simulink model "UrbanPHIL"  (Simulink 8.1)
settings: Solver=ode1  StartTime=0.0  StopTime=inf  FixedStep=Ts  MaxStep=1e-3  RelTol=1e-3
PostLoadFcn:
  | NREL_Mode=1; BANSHEE_init;
InitFcn:
  | NREL_Mode=1; BANSHEE_init;
values from neighbouring files (symbols this model uses):
  Ts = 100E-6    (= 0.0001)    [BANSHEE_init.m]    (also in Ghost_init.m)
undefined symbols (not defined in the file or in its folder): Hydride, Left, Metal, Nickel, type, V
libraries: powerlib x50, rteventslib x26, rtio_opalrt_op5142ex1 x25, artemis x13, simulink x6, cables_lib x4, relay_housing_lib x3, rtlab x2, utility_service_lib x1, Feeder1_lib x1, Feeder2_lib x1, Feeder3_lib x1
(part 3 of 3)

== system UrbanPHIL/SS_PV_BESS/EPC/Inverter_Batt_RTE/TSB_hiZ snubber_free (contains 6 real diode) ==
  note: Rule of the thumb for Rsnubber=Lload/Ts
      | put maximum R for stability,
      | Then add 1-10 uf typ for Csnubber to make sure current goes to zero after a while
  g : Inport
  Demux5 : Demux  Outputs=[2 2 2]
  MMC_1P1 : Subsystem  mask(MMC cell){Ron=1e-3, Vf=0, Gp=1000/100, Gi=100*0.1e-6, Ts=Ts, dc_short_resistance=10, alt_Idc=off, alt_Idc_comp=.5}
      mask prompts: Ron "Switch conduction resistance [Ohms]"; Vf "Switch conduction voltage offset [V]"; Gp "Snubber resistance (in high impedance mode only) [Ohms]"; Gi "Snubber capacitor (in high impedance mode only) [Farads]"; Ts "Sample time [s]"; dc_short_resistance "Anti-voltage reversal equivalent diode resistance  [Ohms]"; alt_Idc "Alternate Idc calculation method based on power balance"; alt_Idc_comp "Alternate Idc compensation factor (default=0) (0...1)"
      mask help:
      | The MMC cell block implement a unipolar bridge with a capacitor.
      | Series RC snubber circuits are connected in parallel with each switch device.
      |
      | Press Help for suggested snubber values when the model is discretized.
      mask Help: eval('fts2help(''ARTEMiSMMC1PCell'');');
      mask Callback alt_Idc:
      | block=gcb;
      | x=get_param(block,'alt_Idc');
      | y=get_param(block,'MaskVisibilities');
      | if isequal (x,'on')
      |     y{8}='on';
      | else
      |     y{8}='off';
      | end
      | set_param(block,'MaskVisibilities',y);
  MMC_1P2 : Subsystem  mask(MMC cell){Ron=1e-3, Vf=0, Gp=1000/100, Gi=100*0.1e-6, Ts=Ts, dc_short_resistance=10, alt_Idc=off, alt_Idc_comp=.5}
      mask prompts: Ron "Switch conduction resistance [Ohms]"; Vf "Switch conduction voltage offset [V]"; Gp "Snubber resistance (in high impedance mode only) [Ohms]"; Gi "Snubber capacitor (in high impedance mode only) [Farads]"; Ts "Sample time [s]"; dc_short_resistance "Anti-voltage reversal equivalent diode resistance  [Ohms]"; alt_Idc "Alternate Idc calculation method based on power balance"; alt_Idc_comp "Alternate Idc compensation factor (default=0) (0...1)"
      mask help:
      | The MMC cell block implement a unipolar bridge with a capacitor.
      | Series RC snubber circuits are connected in parallel with each switch device.
      |
      | Press Help for suggested snubber values when the model is discretized.
      mask Help: eval('fts2help(''ARTEMiSMMC1PCell'');');
      mask Callback alt_Idc:
      | block=gcb;
      | x=get_param(block,'alt_Idc');
      | y=get_param(block,'MaskVisibilities');
      | if isequal (x,'on')
      |     y{8}='on';
      | else
      |     y{8}='off';
      | end
      | set_param(block,'MaskVisibilities',y);
  MMC_1P3 : Subsystem  mask(MMC cell){Ron=1e-3, Vf=0, Gp=1000/100, Gi=100*0.1e-6, Ts=Ts, dc_short_resistance=10, alt_Idc=off, alt_Idc_comp=.5}
      mask prompts: Ron "Switch conduction resistance [Ohms]"; Vf "Switch conduction voltage offset [V]"; Gp "Snubber resistance (in high impedance mode only) [Ohms]"; Gi "Snubber capacitor (in high impedance mode only) [Farads]"; Ts "Sample time [s]"; dc_short_resistance "Anti-voltage reversal equivalent diode resistance  [Ohms]"; alt_Idc "Alternate Idc calculation method based on power balance"; alt_Idc_comp "Alternate Idc compensation factor (default=0) (0...1)"
      mask help:
      | The MMC cell block implement a unipolar bridge with a capacitor.
      | Series RC snubber circuits are connected in parallel with each switch device.
      |
      | Press Help for suggested snubber values when the model is discretized.
      mask Help: eval('fts2help(''ARTEMiSMMC1PCell'');');
      mask Callback alt_Idc:
      | block=gcb;
      | x=get_param(block,'alt_Idc');
      | y=get_param(block,'MaskVisibilities');
      | if isequal (x,'on')
      |     y{8}='on';
      | else
      |     y{8}='off';
      | end
      | set_param(block,'MaskVisibilities',y);
  + : PMIOPort  Port=1  Side=Right
  A : PMIOPort  Port=2  Side=Left
  - : PMIOPort  Port=3  Side=Right
  B : PMIOPort  Port=4  Side=Left
  C : PMIOPort  Port=5  Side=Left
  wires:
  Demux5/1 -> MMC_1P1/1(g)
  Demux5/2 -> MMC_1P2/1(g)
  Demux5/3 -> MMC_1P3/1(g)
  g/1 -> Demux5/1
  connections:
  A/RConn1 -- MMC_1P1/LConn1
  B/RConn1 -- MMC_1P2/LConn1
  C/RConn1 -- MMC_1P3/LConn1
  MMC_1P3/RConn1 -- +/RConn1 -- MMC_1P1/RConn1 -- MMC_1P2/RConn1
  MMC_1P3/RConn2 -- -/RConn1 -- MMC_1P1/RConn2 -- MMC_1P2/RConn2

== system UrbanPHIL/SC_ctrl/EPC Inverter/16TSDIn/16 TSDOut GR3/Dout state ctrl/Dout_CH16_CH23 ==
  Bus Creator1 : BusCreator  Inputs=8
  Dout_CH{16..23} (8 alike) : Constant  Value=[1 0 1 0]
  Manual Switch{17..24} (8 alike) : ManualSwitch
  Zero_Dout_CH{16..23} (8 alike) : Constant  Value=[0 0 0 0]
  Dout_CH8_CH15 : Outport
  wires:
  Bus Creator1/1 -> Dout_CH8_CH15/1
  Dout_CH16/1 -> Manual Switch17/1
  Zero_Dout_CH16/1 -> Manual Switch17/2
  Dout_CH17/1 -> Manual Switch18/1
  Zero_Dout_CH17/1 -> Manual Switch18/2
  Dout_CH18/1 -> Manual Switch19/1
  Zero_Dout_CH18/1 -> Manual Switch19/2
  Dout_CH19/1 -> Manual Switch20/1
  Zero_Dout_CH19/1 -> Manual Switch20/2
  Dout_CH20/1 -> Manual Switch21/1
  Zero_Dout_CH20/1 -> Manual Switch21/2
  Dout_CH21/1 -> Manual Switch22/1
  Zero_Dout_CH21/1 -> Manual Switch22/2
  Dout_CH22/1 -> Manual Switch23/1
  Zero_Dout_CH22/1 -> Manual Switch23/2
  Dout_CH23/1 -> Manual Switch24/1
  Zero_Dout_CH23/1 -> Manual Switch24/2
  Manual Switch17/1 -> Bus Creator1/1  "states 17"
  Manual Switch18/1 -> Bus Creator1/2  "states 18"
  Manual Switch19/1 -> Bus Creator1/3  "states 19"
  Manual Switch20/1 -> Bus Creator1/4  "states 20"
  Manual Switch21/1 -> Bus Creator1/5  "states 21"
  Manual Switch22/1 -> Bus Creator1/6  "states 22"
  Manual Switch23/1 -> Bus Creator1/7  "states 23"
  Manual Switch24/1 -> Bus Creator1/8  "states 24"

== system UrbanPHIL/SC_ctrl/EPC Inverter/16TSDIn/16 TSDOut GR3/Dout state ctrl/Dout_CH24_CH31 ==
  Bus Creator : BusCreator  Inputs=8
  Dout_CH{24..31} (8 alike) : Constant  Value=[1 0 1 0]
  Manual Switch{25..32} (8 alike) : ManualSwitch
  Zero_Dout_CH{24..31} (8 alike) : Constant  Value=[0 0 0 0]
  Dout_CH8_CH15 : Outport
  wires:
  Manual Switch32/1 -> Bus Creator/8  "states 32"
  Manual Switch31/1 -> Bus Creator/7  "states 31"
  Manual Switch30/1 -> Bus Creator/6  "states 30"
  Manual Switch29/1 -> Bus Creator/5  "states 29"
  Manual Switch28/1 -> Bus Creator/4  "states 28"
  Manual Switch27/1 -> Bus Creator/3  "states 27"
  Manual Switch26/1 -> Bus Creator/2  "states 26"
  Manual Switch25/1 -> Bus Creator/1  "states 25"
  Zero_Dout_CH31/1 -> Manual Switch32/2
  Dout_CH31/1 -> Manual Switch32/1
  Zero_Dout_CH30/1 -> Manual Switch31/2
  Dout_CH30/1 -> Manual Switch31/1
  Zero_Dout_CH29/1 -> Manual Switch30/2
  Dout_CH29/1 -> Manual Switch30/1
  Zero_Dout_CH28/1 -> Manual Switch29/2
  Dout_CH28/1 -> Manual Switch29/1
  Zero_Dout_CH27/1 -> Manual Switch28/2
  Dout_CH27/1 -> Manual Switch28/1
  Zero_Dout_CH26/1 -> Manual Switch27/2
  Dout_CH26/1 -> Manual Switch27/1
  Zero_Dout_CH25/1 -> Manual Switch26/2
  Dout_CH25/1 -> Manual Switch26/1
  Zero_Dout_CH24/1 -> Manual Switch25/2
  Dout_CH24/1 -> Manual Switch25/1
  Bus Creator/1 -> Dout_CH8_CH15/1

== system UrbanPHIL/SS_PV_BESS/EPC/Controller Mapping/6-pulse RTE PWM generator (with deadtime)/Discrete Triangular-Waveform Generator ==
  Constant : Constant  Value=Vpeak
  Constant1 : Constant  Value=NumberSteps
  Constant2 : Constant  Value=Freq_used
  Fcn2 : Fcn  Expr=u[2]/u[1]
  Fcn3 : Fcn  Expr=4 *u[1] -1
  Fcn4 : Fcn  Expr=-4 *u[1] +3
  Fd1 : Constant  Value=-1
  Fd2 : Constant
  Fd4 : Constant
  Gain1 : Gain  Gain=1/2  SaturateOnIntegerOverflow=on  OutDataTypeStr=Inherit: Same as input  ParamDataTypeStr=Inherit: Same as input
  Mux5 : Mux  Inputs=2
  Product : Product  SaturateOnIntegerOverflow=on  InputSameDT=on  OutDataTypeStr=Inherit: Same as first input
  Relational Operator1 : RelationalOperator  Operator=>  InputSameDT=on
  Relational Operator2 : RelationalOperator  Operator===  InputSameDT=on
  Sum : Sum  SaturateOnIntegerOverflow=on  InputSameDT=on  OutDataTypeStr=Inherit: Same as first input
  Sum2 : Sum  Inputs=+-  SaturateOnIntegerOverflow=on  InputSameDT=on  OutDataTypeStr=Inherit: Same as first input
  Switch : Switch  Threshold=0.5  SaturateOnIntegerOverflow=on  InputSameDT=on
  Switch1 : Switch  Threshold=0.5  SaturateOnIntegerOverflow=on  InputSameDT=on
  Unit Delay : UnitDelay  SampleTime=Ts
  Unit Delay1 : UnitDelay  SampleTime=Ts
  Triangle : Outport  InitialOutput=0
  Freq_used : Outport  Port=2  InitialOutput=0
  wires:
  Constant2/1 -> Freq_used/1
  Relational Operator1/1 -> Switch1/2
  Gain1/1 -> Relational Operator1/2
  Fcn3/1 -> Switch1/3
  Fcn4/1 -> Switch1/1
  Mux5/1 -> Fcn2/1
  Fcn2/1 -> Fcn3/1, Fcn4/1
  Sum/1 -> Mux5/2, Relational Operator1/1, Relational Operator2/2, Unit Delay/1
  Constant1/1 -> Gain1/1, Mux5/1, Sum2/1
  Sum2/1 -> Relational Operator2/1
  Relational Operator2/1 -> Unit Delay1/1
  Unit Delay1/1 -> Switch/2
  Unit Delay/1 -> Switch/3
  Fd1/1 -> Switch/1
  Fd2/1 -> Sum/2
  Switch/1 -> Sum/1
  Fd4/1 -> Sum2/2
  Constant/1 -> Product/1
  Switch1/1 -> Product/2
  Product/1 -> Triangle/1

== system UrbanPHIL/SS_PV_BESS/EPC/Controller Mapping/EPC Inverter Controller Outputs/DIO - Gr4 ==
  Dout : Inport
  Bus Creator : BusCreator  Inputs=2
  Bus Selector : BusSelector  OutputSignals=DI_CH00-07  OutputAsBus=on
  Bus Selector1 : BusSelector  OutputSignals=DI_CH08-15  OutputAsBus=on
  Conditioning : Subsystem
  Conditioning1 : Subsystem
  OP5142EX2 DigitalIn : rtio_opalrt_op5142ex1/OP5142EX1 DigitalIn  CtrlName='OP5142EX2 Ctrl'  portNb=3  FcnNos=Slot 4 Module A Subsection 1  size=1  maxcount=8  count=8  sampleTime=0  numchan=8
      settings: AttributesFormatString=%<CtrlName>
  OP5142EX2 DigitalIn1 : rtio_opalrt_op5142ex1/OP5142EX1 DigitalIn  CtrlName='OP5142EX2 Ctrl'  portNb=4  FcnNos=Slot 4 Module A Subsection 2  size=1  maxcount=8  count=8  sampleTime=0  numchan=8
      settings: AttributesFormatString=%<CtrlName>
  OP5142EX2 DigitalOut : rtio_opalrt_op5142ex1/OP5142EX1 DigitalOut  CtrlName='OP5142EX2 Ctrl'  portNb=9  FcnNos=Slot 4 Module B Subsection 1  size=1  maxcount=8  count=8  numchan=8
      settings: AttributesFormatString=%<CtrlName>
  OP5142EX2 DigitalOut1 : rtio_opalrt_op5142ex1/OP5142EX1 DigitalOut  CtrlName='OP5142EX2 Ctrl'  portNb=10  FcnNos=Slot 4 Module B Subsection 2  size=1  maxcount=8  count=8  numchan=8
      settings: AttributesFormatString=%<CtrlName>
  Terminator{1,3,5..6} (4 alike) : Terminator
  DIn : Outport
  wires:
  OP5142EX2 DigitalOut/1 -> Terminator3/1
  OP5142EX2 DigitalOut1/1 -> Terminator1/1
  Dout/1 -> Bus Selector/1, Bus Selector1/1
  Bus Selector/1 -> OP5142EX2 DigitalOut/1
  Bus Selector1/1 -> OP5142EX2 DigitalOut1/1
  OP5142EX2 DigitalIn/2 -> Terminator5/1
  OP5142EX2 DigitalIn1/2 -> Terminator6/1
  OP5142EX2 DigitalIn/1 -> Conditioning/1(In1)  "DI_CH00-07"
  OP5142EX2 DigitalIn1/1 -> Conditioning1/1(In1)  "DI_CH08-15"
  Bus Creator/1 -> DIn/1
  Conditioning/1(Out1) -> Bus Creator/1
  Conditioning1/1(Out1) -> Bus Creator/2

== system UrbanPHIL/SS_PV_BESS/EPC/Controller Mapping/EPC Inverter Controller Outputs/DOUT type config ==
  note: The Constants are used to select Digital Output type:
      | - 0: Time-Stamped Digital Output
      | - 1: Pulse-Width Modulated DIgital Output
  OP5142EX2 DataIn Send : rtio_opalrt_op5142ex1/OP5142EX1 DataIn Send  CtrlName='OP5142EX2 Ctrl'  FcnNosp1=15  FcnNos=-1  FcnNosm1=(15)-1  width=1  portType=double  numwidth=1
      settings: AttributesFormatString=%<CtrlName>
  OP5142EX2 DataIn Send1 : rtio_opalrt_op5142ex1/OP5142EX1 DataIn Send  CtrlName='OP5142EX2 Ctrl'  FcnNosp1=16  FcnNos=-1  FcnNosm1=(16)-1  width=1  portType=double  numwidth=1
      settings: AttributesFormatString=%<CtrlName>
  Subsection 3 DOUT type : Constant  Value=0
  Subsection 4 DOUT type : Constant  Value=0
  Terminator1 : Terminator
  Terminator2 : Terminator
  wires:
  Subsection 3 DOUT type/1 -> OP5142EX2 DataIn Send/1
  Subsection 4 DOUT type/1 -> OP5142EX2 DataIn Send1/1
  OP5142EX2 DataIn Send1/1 -> Terminator1/1
  OP5142EX2 DataIn Send/1 -> Terminator2/1

== system UrbanPHIL/SS_PV_BESS/EPC/Controller Mapping/EPC Inverter Controller Outputs/GR1 B AIN (CH00-15) ==
  Mux6 : Mux  Inputs=2
  OP5142EX2 AnalogIn : rtio_opalrt_op5142ex1/OP5142EX1 AnalogIn  CtrlName='OP5142EX2 Ctrl'  portNb=1  FcnNos=Slot 1 Module B Subsection 1  size=16  maxcount=8  count=8  numchan=8  sampleTime=0
      settings: AttributesFormatString=%<CtrlName>
  OP5142EX2 AnalogIn1 : rtio_opalrt_op5142ex1/OP5142EX1 AnalogIn  CtrlName='OP5142EX2 Ctrl'  portNb=2  FcnNos=Slot 1 Module B Subsection 2  size=16  maxcount=8  count=8  numchan=8  sampleTime=0
      settings: AttributesFormatString=%<CtrlName>
  Terminator2 : Terminator
  Terminator3 : Terminator
  Ain : Outport
  wires:
  Mux6/1 -> Ain/1
  OP5142EX2 AnalogIn1/2 -> Terminator3/1
  OP5142EX2 AnalogIn/2 -> Terminator2/1
  OP5142EX2 AnalogIn1/1 -> Mux6/2
  OP5142EX2 AnalogIn/1 -> Mux6/1

== system UrbanPHIL/SS_PV_BESS/EPC/Controller Mapping/EPC Inverter Controller Outputs/PWM IO - Gr4 ==
  PWMOut : Inport
  Bus Creator : BusCreator  Inputs=2
  Bus Creator1 : BusCreator  Inputs=2
  Bus Creator2 : BusCreator  Inputs=2
  Bus Selector : BusSelector  OutputSignals=FreqPWMOut16-23,DutyPWMOut16-23
  Bus Selector1 : BusSelector  OutputSignals=FreqPWMOut24-31,DutyPWMOut24-31
  Bus Selector2 : BusSelector  OutputSignals=Ch16-23,Ch24-31
  OP5142EX2 PWM In : rtio_opalrt_op5142ex1/OP5142EX1 PWM In  CtrlName='OP5142EX2 Ctrl'  portNb=7  FcnNos=Slot 4 Module A Subsection 3  maxCount=8  Count=8  sampleTime=0  numchan=8
      settings: AttributesFormatString=%<CtrlName>
  OP5142EX2 PWM In1 : rtio_opalrt_op5142ex1/OP5142EX1 PWM In  CtrlName='OP5142EX2 Ctrl'  portNb=8  FcnNos=Slot 4 Module A Subsection 4  maxCount=8  Count=8  sampleTime=0  numchan=8
      settings: AttributesFormatString=%<CtrlName>
  OP5142EX2 PWM Out : rtio_opalrt_op5142ex1/OP5142EX1 PWM Out  CtrlName='OP5142EX2 Ctrl'  portNb=13  FcnNos=Slot 4 Module B Subsection 3  size=64  maxcount=8  count=8  polarity=Active High  symMode=Symmetric  complementary=off  deadTime=0  numchan=8  loadnb=1  initphase=[0 0 0 0 0 0 0 0]  dutyhalf=At each PWM period
      settings: AttributesFormatString=%<CtrlName>
  OP5142EX2 PWM Out1 : rtio_opalrt_op5142ex1/OP5142EX1 PWM Out  CtrlName='OP5142EX2 Ctrl'  portNb=14  FcnNos=Slot 4 Module B Subsection 4  size=64  maxcount=8  count=8  polarity=Active High  symMode=Symmetric  complementary=off  deadTime=0  numchan=8  loadnb=2  initphase=[0 0 0 0 0 0 0 0]  dutyhalf=At each PWM period
      settings: AttributesFormatString=%<CtrlName>
  RTE PWM Top 1 : rteventslib/Sources/RTE PWM  ShiftedTransition=Enabled  MaxEvents=4  SampleTime=Ts
  Terminator{,1,4..5} (4 alike) : Terminator
  PWMIn : Outport
  PWMIn_RTE : Outport  Port=2
  wires:
  Bus Selector/1 -> OP5142EX2 PWM Out/1  "<FreqPWMOut16-23>"
  Bus Selector/2 -> OP5142EX2 PWM Out/2  "<DutyPWMOut16-23>"
  OP5142EX2 PWM Out/1 -> Terminator/1
  Bus Selector1/1 -> OP5142EX2 PWM Out1/1  "<FreqPWMOut24-31>"
  Bus Selector1/2 -> OP5142EX2 PWM Out1/2  "<DutyPWMOut24-31>"
  OP5142EX2 PWM Out1/1 -> Terminator1/1
  PWMOut/1 -> Bus Selector2/1
  Bus Selector2/1 -> Bus Selector/1  "<Ch16-23>"
  Bus Creator/1 -> PWMIn/1
  Bus Creator1/1 -> Bus Creator/1  "PWMI_CH16-23"
  Bus Creator2/1 -> Bus Creator/2  "PWMI_CH24-31"
  OP5142EX2 PWM In1/3 -> Terminator5/1
  OP5142EX2 PWM In/3 -> Terminator4/1
  OP5142EX2 PWM In/1 -> Bus Creator1/1, RTE PWM Top 1/1  "Freq"
  OP5142EX2 PWM In/2 -> Bus Creator1/2, RTE PWM Top 1/2  "Duty"
  OP5142EX2 PWM In1/1 -> Bus Creator2/1  "Freq"
  OP5142EX2 PWM In1/2 -> Bus Creator2/2  "Duty"
  Bus Selector2/2 -> Bus Selector1/1  "<Ch24-31>"
  RTE PWM Top 1/1 -> PWMIn_RTE/1

== system UrbanPHIL/SS_PV_BESS/EPC/Controller Mapping/EPC Inverter Controller Outputs/TSDIO - Gr4 ==
  note: States
      | Times
      | for each channel
      |
      | Status for the block.
  TSDout : Inport
  Bus Creator : BusCreator  Inputs=16
  Bus Creator1 : BusCreator  Inputs=16
  Bus Creator2 : BusCreator  Inputs=2
  Bus Selector : BusSelector  OutputSignals=states.CH16-23.states 17,times CH16-23.times17,states.CH16-23.states 18,times CH16-23.times18,states.CH16-23.states 19,times CH16-23.times19,states.CH16-23.states 20,times CH16-23.times20,states.CH16-23.states 21,times CH16-23.times21,states.CH16-23.states 22,times CH16-23.times22,states.CH16-23.states 23,times CH16-23.times23,states.CH16-23.states 24,times CH16-23.times24
  Bus Selector1 : BusSelector  OutputSignals=states.CH24-31.states 25,times CH24-31.times25,states.CH24-31.states 26,times CH24-31.times26,states.CH24-31.states 27,times CH24-31.times27,states.CH24-31.states 28,times CH24-31.times28,states.CH24-31.states 29,times CH24-31.times29,states.CH24-31.states 30,times CH24-31.times30,states.CH24-31.states 31,times CH24-31.times31,states.CH24-31.states 32,times CH24-31.times32
  Bus Selector2 : BusSelector  OutputSignals=states1,times1,states2,times2,states3,times3,states4,times4,states5,times5,states6,times6
  OP5142EX2 EventDetector : rtio_opalrt_op5142ex1/OP5142EX1 EventDetector  CtrlName='OP5142EX2 Ctrl'  portNb=5  FcnNos=Slot 4 Module A Subsection 3  size=32  count=8  nbChannels=8  width=4  timeUnit=Time ratio  sampleTime=0  numwidth=4
      settings: AttributesFormatString=%<CtrlName>
  OP5142EX2 EventDetector1 : rtio_opalrt_op5142ex1/OP5142EX1 EventDetector  CtrlName='OP5142EX2 Ctrl'  portNb=6  FcnNos=Slot 4 Module A Subsection 4  size=32  count=8  nbChannels=8  width=4  timeUnit=Time ratio  sampleTime=0  numwidth=4
      settings: AttributesFormatString=%<CtrlName>
  OP5142EX2 EventGenerator : rtio_opalrt_op5142ex1/OP5142EX1 EventGenerator  CtrlName='OP5142EX2 Ctrl'  portNb=11  FcnNos=Slot 4 Module B Subsection 3  size=32  count=8  nbChannels=8  width=4  timeUnit=Time ratio  numwidth=4
      settings: AttributesFormatString=%<CtrlName>
  OP5142EX2 EventGenerator1 : rtio_opalrt_op5142ex1/OP5142EX1 EventGenerator  CtrlName='OP5142EX2 Ctrl'  portNb=12  FcnNos=Slot 4 Module B Subsection 4  size=32  count=8  nbChannels=8  width=4  timeUnit=Time ratio  numwidth=4
      settings: AttributesFormatString=%<CtrlName>
  RTE Conversion OP5110-5120 Event Generator/Detector : rteventslib/Signal Attributes/RTE Conversion OP5110-5120 Event Generator//Detector  conversionType=OP5110-5120 to RTE Boolean  nbLine=6  nbEvents=4  timeUnit=Time Ratio  enTimeFactor=off  sampleTime=Ts  initStates=off
  Terminator{,1..3} (4 alike) : Terminator
  TSDin : Outport
  TSDin_RTE : Outport  Port=2
  wires:
  TSDout/1 -> Bus Selector/1, Bus Selector1/1
  Bus Selector/16 -> OP5142EX2 EventGenerator/16  "<times24>"
  Bus Selector/15 -> OP5142EX2 EventGenerator/15  "<states 24>"
  Bus Selector/14 -> OP5142EX2 EventGenerator/14  "<times23>"
  Bus Selector/13 -> OP5142EX2 EventGenerator/13  "<states 23>"
  Bus Selector/12 -> OP5142EX2 EventGenerator/12  "<times22>"
  Bus Selector/11 -> OP5142EX2 EventGenerator/11  "<states 22>"
  Bus Selector/10 -> OP5142EX2 EventGenerator/10  "<times21>"
  Bus Selector/9 -> OP5142EX2 EventGenerator/9  "<states 21>"
  Bus Selector/8 -> OP5142EX2 EventGenerator/8  "<times20>"
  Bus Selector/7 -> OP5142EX2 EventGenerator/7  "<states 20>"
  Bus Selector/6 -> OP5142EX2 EventGenerator/6  "<times19>"
  Bus Selector/5 -> OP5142EX2 EventGenerator/5  "<states 19>"
  Bus Selector/4 -> OP5142EX2 EventGenerator/4  "<times18>"
  Bus Selector/3 -> OP5142EX2 EventGenerator/3  "<states 18>"
  Bus Selector/2 -> OP5142EX2 EventGenerator/2  "<times17>"
  Bus Selector/1 -> OP5142EX2 EventGenerator/1  "<states 17>"
  OP5142EX2 EventGenerator/1 -> Terminator/1
  OP5142EX2 EventDetector/16 -> Bus Creator/16  "times8"
  OP5142EX2 EventDetector/15 -> Bus Creator/15  "states8"
  OP5142EX2 EventDetector/14 -> Bus Creator/14  "times7"
  OP5142EX2 EventDetector/13 -> Bus Creator/13  "states7"
  OP5142EX2 EventDetector/12 -> Bus Creator/12  "times6"
  OP5142EX2 EventDetector/11 -> Bus Creator/11  "states6"
  OP5142EX2 EventDetector/10 -> Bus Creator/10  "times5"
  OP5142EX2 EventDetector/9 -> Bus Creator/9  "states5"
  OP5142EX2 EventDetector/8 -> Bus Creator/8  "times4"
  OP5142EX2 EventDetector/7 -> Bus Creator/7  "states4"
  OP5142EX2 EventDetector/6 -> Bus Creator/6  "times3"
  OP5142EX2 EventDetector/5 -> Bus Creator/5  "states3"
  OP5142EX2 EventDetector/4 -> Bus Creator/4  "times2"
  OP5142EX2 EventDetector/3 -> Bus Creator/3  "states2"
  OP5142EX2 EventDetector/2 -> Bus Creator/2  "times1"
  OP5142EX2 EventDetector/1 -> Bus Creator/1  "states1"
  OP5142EX2 EventDetector/17 -> Terminator1/1, [status]
  OP5142EX2 EventGenerator1/1 -> Terminator2/1
  Bus Selector1/1 -> OP5142EX2 EventGenerator1/1  "<states 25>"
  Bus Selector1/2 -> OP5142EX2 EventGenerator1/2  "<times25>"
  Bus Selector1/3 -> OP5142EX2 EventGenerator1/3  "<states 26>"
  Bus Selector1/4 -> OP5142EX2 EventGenerator1/4  "<times26>"
  Bus Selector1/5 -> OP5142EX2 EventGenerator1/5  "<states 27>"
  Bus Selector1/6 -> OP5142EX2 EventGenerator1/6  "<times27>"
  Bus Selector1/7 -> OP5142EX2 EventGenerator1/7  "<states 28>"
  Bus Selector1/8 -> OP5142EX2 EventGenerator1/8  "<times28>"
  Bus Selector1/9 -> OP5142EX2 EventGenerator1/9  "<states 29>"
  Bus Selector1/10 -> OP5142EX2 EventGenerator1/10  "<times29>"
  Bus Selector1/11 -> OP5142EX2 EventGenerator1/11  "<states 30>"
  Bus Selector1/12 -> OP5142EX2 EventGenerator1/12  "<times30>"
  Bus Selector1/13 -> OP5142EX2 EventGenerator1/13  "<states 31>"
  Bus Selector1/14 -> OP5142EX2 EventGenerator1/14  "<times31>"
  Bus Selector1/15 -> OP5142EX2 EventGenerator1/15  "<states 32>"
  Bus Selector1/16 -> OP5142EX2 EventGenerator1/16  "<times32>"
  Bus Creator1/1 -> Bus Creator2/2  "CH24-31"
  OP5142EX2 EventDetector1/16 -> Bus Creator1/16  "times6"
  OP5142EX2 EventDetector1/15 -> Bus Creator1/15  "states6"
  OP5142EX2 EventDetector1/14 -> Bus Creator1/14  "times5"
  OP5142EX2 EventDetector1/13 -> Bus Creator1/13  "states5"
  OP5142EX2 EventDetector1/12 -> Bus Creator1/12  "times4"
  OP5142EX2 EventDetector1/11 -> Bus Creator1/11  "states4"
  OP5142EX2 EventDetector1/10 -> Bus Creator1/10  "times3"
  OP5142EX2 EventDetector1/9 -> Bus Creator1/9  "states3"
  OP5142EX2 EventDetector1/8 -> Bus Creator1/8  "times2"
  OP5142EX2 EventDetector1/7 -> Bus Creator1/7  "states2"
  OP5142EX2 EventDetector1/6 -> Bus Creator1/6  "times1"
  OP5142EX2 EventDetector1/5 -> Bus Creator1/5  "states1"
  OP5142EX2 EventDetector1/4 -> Bus Creator1/4  "times2"
  OP5142EX2 EventDetector1/3 -> Bus Creator1/3  "states2"
  OP5142EX2 EventDetector1/2 -> Bus Creator1/2  "times1"
  OP5142EX2 EventDetector1/1 -> Bus Creator1/1  "states1"
  OP5142EX2 EventDetector1/17 -> Terminator3/1  "states7"
  Bus Creator/1 -> Bus Creator2/1, Bus Selector2/1  "CH16-23"
  Bus Creator2/1 -> TSDin/1  "TSDIN"
  Bus Selector2/1 -> RTE Conversion OP5110-5120 Event Generator/Detector/1  "<states1>"
  Bus Selector2/3 -> RTE Conversion OP5110-5120 Event Generator/Detector/4  "<states2>"
  [status] -> RTE Conversion OP5110-5120 Event Generator/Detector/3
  [status] -> RTE Conversion OP5110-5120 Event Generator/Detector/6
  Bus Selector2/5 -> RTE Conversion OP5110-5120 Event Generator/Detector/7  "<states3>"
  Bus Selector2/2 -> RTE Conversion OP5110-5120 Event Generator/Detector/2  "<times1>"
  Bus Selector2/4 -> RTE Conversion OP5110-5120 Event Generator/Detector/5  "<times2>"
  Bus Selector2/6 -> RTE Conversion OP5110-5120 Event Generator/Detector/8  "<times3>"
  [status] -> RTE Conversion OP5110-5120 Event Generator/Detector/9
  Bus Selector2/7 -> RTE Conversion OP5110-5120 Event Generator/Detector/10  "<states4>"
  Bus Selector2/8 -> RTE Conversion OP5110-5120 Event Generator/Detector/11  "<times4>"
  [status] -> RTE Conversion OP5110-5120 Event Generator/Detector/12
  Bus Selector2/9 -> RTE Conversion OP5110-5120 Event Generator/Detector/13  "<states5>"
  Bus Selector2/10 -> RTE Conversion OP5110-5120 Event Generator/Detector/14  "<times5>"
  [status] -> RTE Conversion OP5110-5120 Event Generator/Detector/15
  Bus Selector2/11 -> RTE Conversion OP5110-5120 Event Generator/Detector/16  "<states6>"
  Bus Selector2/12 -> RTE Conversion OP5110-5120 Event Generator/Detector/17  "<times6>"
  [status] -> RTE Conversion OP5110-5120 Event Generator/Detector/18
  RTE Conversion OP5110-5120 Event Generator/Detector/1 -> TSDin_RTE/1

== system UrbanPHIL/SS_PV_BESS/EPC/Inverter_Batt_RTE/TSB_hiZ snubber_free (contains 6 real diode)/MMC_1P1 ==
  g : Inport
  Constant2 : Constant  Value=Ts
  Constant9 : Constant  Value=0
  Controlled Current Source : powerlib/Electrical Sources/Controlled Current Source  Initialize=on  Source_Type=AC  Amplitude=0  Phase=0  Frequency=0  Measurements=None
  Demux1 : Demux  Outputs=2
  Diode : powerlib/Power Electronics/Diode  Ron=Ron  Lon=0  Vf=0  IC=0  UseSnubber=off  Rs=Gp  Cs=Gi  Measurements=off
  Diode1 : powerlib/Power Electronics/Diode  Ron=Ron  Lon=0  Vf=0  IC=0  UseSnubber=off  Rs=Gp  Cs=Gi  Measurements=off
  IMeasure_1 : powerlib/Measurements/Current Measurement  PhasorSimulation=off  OutputType=Magnitude  PSBequivalent=0
  IMeasure_2 : powerlib/Measurements/Current Measurement  PhasorSimulation=off  OutputType=Magnitude  PSBequivalent=0
  MMC_cell_Sfunction : Subsystem
  Memory1 : Memory  InheritSampleTime=on
  Memory2 : Memory  InheritSampleTime=on
  Memory4 : Memory  InheritSampleTime=on
  Switch1 : Switch  Threshold=0.5
  Switch2 : Switch  Threshold=0.5
  Switch4 : Switch  Threshold=0.5
  VSource_2 : powerlib/Electrical Sources/Controlled Voltage Source  Initialize=off  Source_Type=AC  Amplitude=0  Phase=0  Frequency=0  Measurements=None
  VSource_3 : powerlib/Electrical Sources/Controlled Voltage Source  Initialize=off  Source_Type=AC  Amplitude=0  Phase=0  Frequency=0  Measurements=None
  Voltage Measurement : powerlib/Measurements/Voltage Measurement  PhasorSimulation=off  OutputType=Complex  PSBequivalent=0
  A : PMIOPort  Port=1  Side=Left
  Dc+ : PMIOPort  Port=2  Side=Right
  Dc- : PMIOPort  Port=3  Side=Right
  wires:
  g/1 -> Demux1/1
  Demux1/2 -> MMC_cell_Sfunction/2(g1)
  Demux1/1 -> MMC_cell_Sfunction/1(g)
  Constant2/1 -> MMC_cell_Sfunction/3(Ts)
  MMC_cell_Sfunction/2(Vac) -> Switch4/3, Switch1/3
  IMeasure_1/1 -> Memory1/1
  Voltage Measurement/1 -> Memory4/1
  Switch4/1 -> VSource_2/1
  Switch1/1 -> VSource_3/1
  MMC_cell_Sfunction/3(hiZ) -> Switch4/2, Switch1/2, Switch2/2
  Constant9/1 -> Switch4/1
  Memory1/1 -> MMC_cell_Sfunction/4(Iac)
  Memory4/1 -> MMC_cell_Sfunction/5(Vdc), Switch1/1
  Switch2/1 -> Controlled Current Source/1
  MMC_cell_Sfunction/1(Idc) -> Switch2/3
  IMeasure_2/1 -> Memory2/1
  Memory2/1 -> Switch2/1
  connections:
  Controlled Current Source/RConn1 -- Dc-/RConn1 -- Voltage Measurement/LConn2 -- VSource_3/LConn1 -- VSource_2/LConn1
  Dc+/RConn1 -- Voltage Measurement/LConn1 -- Controlled Current Source/LConn1
  Diode1/LConn1 -- VSource_2/RConn1
  Diode1/RConn1 -- Diode/LConn1 -- IMeasure_1/LConn1
  IMeasure_1/RConn1 -- A/RConn1
  VSource_3/RConn1 -- IMeasure_2/LConn1
  IMeasure_2/RConn1 -- Diode/RConn1

== system UrbanPHIL/SS_PV_BESS/EPC/Inverter_Batt_RTE/TSB_hiZ snubber_free (contains 6 real diode)/MMC_1P2 ==
  g : Inport
  Constant2 : Constant  Value=Ts
  Constant9 : Constant  Value=0
  Controlled Current Source : powerlib/Electrical Sources/Controlled Current Source  Initialize=on  Source_Type=AC  Amplitude=0  Phase=0  Frequency=0  Measurements=None
  Demux1 : Demux  Outputs=2
  Diode : powerlib/Power Electronics/Diode  Ron=Ron  Lon=0  Vf=0  IC=0  UseSnubber=off  Rs=Gp  Cs=Gi  Measurements=off
  Diode1 : powerlib/Power Electronics/Diode  Ron=Ron  Lon=0  Vf=0  IC=0  UseSnubber=off  Rs=Gp  Cs=Gi  Measurements=off
  IMeasure_1 : powerlib/Measurements/Current Measurement  PhasorSimulation=off  OutputType=Magnitude  PSBequivalent=0
  IMeasure_2 : powerlib/Measurements/Current Measurement  PhasorSimulation=off  OutputType=Magnitude  PSBequivalent=0
  MMC_cell_Sfunction : Subsystem
  Memory1 : Memory  InheritSampleTime=on
  Memory2 : Memory  InheritSampleTime=on
  Memory4 : Memory  InheritSampleTime=on
  Switch1 : Switch  Threshold=0.5
  Switch2 : Switch  Threshold=0.5
  Switch4 : Switch  Threshold=0.5
  VSource_2 : powerlib/Electrical Sources/Controlled Voltage Source  Initialize=off  Source_Type=AC  Amplitude=0  Phase=0  Frequency=0  Measurements=None
  VSource_3 : powerlib/Electrical Sources/Controlled Voltage Source  Initialize=off  Source_Type=AC  Amplitude=0  Phase=0  Frequency=0  Measurements=None
  Voltage Measurement : powerlib/Measurements/Voltage Measurement  PhasorSimulation=off  OutputType=Complex  PSBequivalent=0
  A : PMIOPort  Port=1  Side=Left
  Dc+ : PMIOPort  Port=2  Side=Right
  Dc- : PMIOPort  Port=3  Side=Right
  wires:
  Memory2/1 -> Switch2/1
  IMeasure_2/1 -> Memory2/1
  MMC_cell_Sfunction/1(Idc) -> Switch2/3
  Switch2/1 -> Controlled Current Source/1
  Memory4/1 -> Switch1/1, MMC_cell_Sfunction/5(Vdc)
  Memory1/1 -> MMC_cell_Sfunction/4(Iac)
  Constant9/1 -> Switch4/1
  MMC_cell_Sfunction/3(hiZ) -> Switch2/2, Switch1/2, Switch4/2
  Switch1/1 -> VSource_3/1
  Switch4/1 -> VSource_2/1
  Voltage Measurement/1 -> Memory4/1
  IMeasure_1/1 -> Memory1/1
  MMC_cell_Sfunction/2(Vac) -> Switch1/3, Switch4/3
  Constant2/1 -> MMC_cell_Sfunction/3(Ts)
  Demux1/1 -> MMC_cell_Sfunction/1(g)
  Demux1/2 -> MMC_cell_Sfunction/2(g1)
  g/1 -> Demux1/1
  connections:
  IMeasure_2/RConn1 -- Diode/RConn1
  VSource_3/RConn1 -- IMeasure_2/LConn1
  IMeasure_1/RConn1 -- A/RConn1
  IMeasure_1/LConn1 -- Diode/LConn1 -- Diode1/RConn1
  Diode1/LConn1 -- VSource_2/RConn1
  Controlled Current Source/LConn1 -- Voltage Measurement/LConn1 -- Dc+/RConn1
  VSource_2/LConn1 -- VSource_3/LConn1 -- Voltage Measurement/LConn2 -- Dc-/RConn1 -- Controlled Current Source/RConn1

== system UrbanPHIL/SS_PV_BESS/EPC/Inverter_Batt_RTE/TSB_hiZ snubber_free (contains 6 real diode)/MMC_1P3 ==
  g : Inport
  Constant2 : Constant  Value=Ts
  Constant9 : Constant  Value=0
  Controlled Current Source : powerlib/Electrical Sources/Controlled Current Source  Initialize=on  Source_Type=AC  Amplitude=0  Phase=0  Frequency=0  Measurements=None
  Demux1 : Demux  Outputs=2
  Diode : powerlib/Power Electronics/Diode  Ron=Ron  Lon=0  Vf=0  IC=0  UseSnubber=off  Rs=Gp  Cs=Gi  Measurements=off
  Diode1 : powerlib/Power Electronics/Diode  Ron=Ron  Lon=0  Vf=0  IC=0  UseSnubber=off  Rs=Gp  Cs=Gi  Measurements=off
  IMeasure_1 : powerlib/Measurements/Current Measurement  PhasorSimulation=off  OutputType=Magnitude  PSBequivalent=0
  IMeasure_2 : powerlib/Measurements/Current Measurement  PhasorSimulation=off  OutputType=Magnitude  PSBequivalent=0
  MMC_cell_Sfunction : Subsystem
  Memory1 : Memory  InheritSampleTime=on
  Memory2 : Memory  InheritSampleTime=on
  Memory4 : Memory  InheritSampleTime=on
  Switch1 : Switch  Threshold=0.5
  Switch2 : Switch  Threshold=0.5
  Switch4 : Switch  Threshold=0.5
  VSource_2 : powerlib/Electrical Sources/Controlled Voltage Source  Initialize=off  Source_Type=AC  Amplitude=0  Phase=0  Frequency=0  Measurements=None
  VSource_3 : powerlib/Electrical Sources/Controlled Voltage Source  Initialize=off  Source_Type=AC  Amplitude=0  Phase=0  Frequency=0  Measurements=None
  Voltage Measurement : powerlib/Measurements/Voltage Measurement  PhasorSimulation=off  OutputType=Complex  PSBequivalent=0
  A : PMIOPort  Port=1  Side=Left
  Dc+ : PMIOPort  Port=2  Side=Right
  Dc- : PMIOPort  Port=3  Side=Right
  wires:
  g/1 -> Demux1/1
  Demux1/2 -> MMC_cell_Sfunction/2(g1)
  Demux1/1 -> MMC_cell_Sfunction/1(g)
  Constant2/1 -> MMC_cell_Sfunction/3(Ts)
  MMC_cell_Sfunction/2(Vac) -> Switch4/3, Switch1/3
  IMeasure_1/1 -> Memory1/1
  Voltage Measurement/1 -> Memory4/1
  Switch4/1 -> VSource_2/1
  Switch1/1 -> VSource_3/1
  MMC_cell_Sfunction/3(hiZ) -> Switch4/2, Switch1/2, Switch2/2
  Constant9/1 -> Switch4/1
  Memory1/1 -> MMC_cell_Sfunction/4(Iac)
  Memory4/1 -> MMC_cell_Sfunction/5(Vdc), Switch1/1
  Switch2/1 -> Controlled Current Source/1
  MMC_cell_Sfunction/1(Idc) -> Switch2/3
  IMeasure_2/1 -> Memory2/1
  Memory2/1 -> Switch2/1
  connections:
  Controlled Current Source/RConn1 -- Dc-/RConn1 -- Voltage Measurement/LConn2 -- VSource_3/LConn1 -- VSource_2/LConn1
  Dc+/RConn1 -- Voltage Measurement/LConn1 -- Controlled Current Source/LConn1
  Diode1/LConn1 -- VSource_2/RConn1
  Diode1/RConn1 -- Diode/LConn1 -- IMeasure_1/LConn1
  IMeasure_1/RConn1 -- A/RConn1
  VSource_3/RConn1 -- IMeasure_2/LConn1
  IMeasure_2/RConn1 -- Diode/RConn1

== system UrbanPHIL/SS_PV_BESS/EPC/Controller Mapping/EPC Inverter Controller Outputs/DIO - Gr4/Conditioning ==
  In1 : Inport
  Bus Creator : BusCreator  Inputs=8
  Demux : Demux  Outputs=8
  Out1 : Outport
  wires:
  Demux/1 -> Bus Creator/1  "K2_Main_DC"
  Demux/2 -> Bus Creator/2  "K1_Precharge_DC"
  Demux/3 -> Bus Creator/3  "MX2_Remote_AC"
  Demux/4 -> Bus Creator/4  "MX1_Main_AC"
  Demux/5 -> Bus Creator/5
  Demux/6 -> Bus Creator/6
  Demux/7 -> Bus Creator/7
  Demux/8 -> Bus Creator/8
  Bus Creator/1 -> Out1/1  "DI_CH00-07"
  In1/1 -> Demux/1

== system UrbanPHIL/SS_PV_BESS/EPC/Controller Mapping/EPC Inverter Controller Outputs/DIO - Gr4/Conditioning1 ==
  In1 : Inport
  Bus Creator : BusCreator  Inputs=8
  Demux : Demux  Outputs=8
  Out1 : Outport
  wires:
  In1/1 -> Demux/1
  Bus Creator/1 -> Out1/1  "DI_CH08-15"
  Demux/8 -> Bus Creator/8
  Demux/7 -> Bus Creator/7
  Demux/6 -> Bus Creator/6
  Demux/5 -> Bus Creator/5
  Demux/4 -> Bus Creator/4
  Demux/3 -> Bus Creator/3
  Demux/2 -> Bus Creator/2
  Demux/1 -> Bus Creator/1

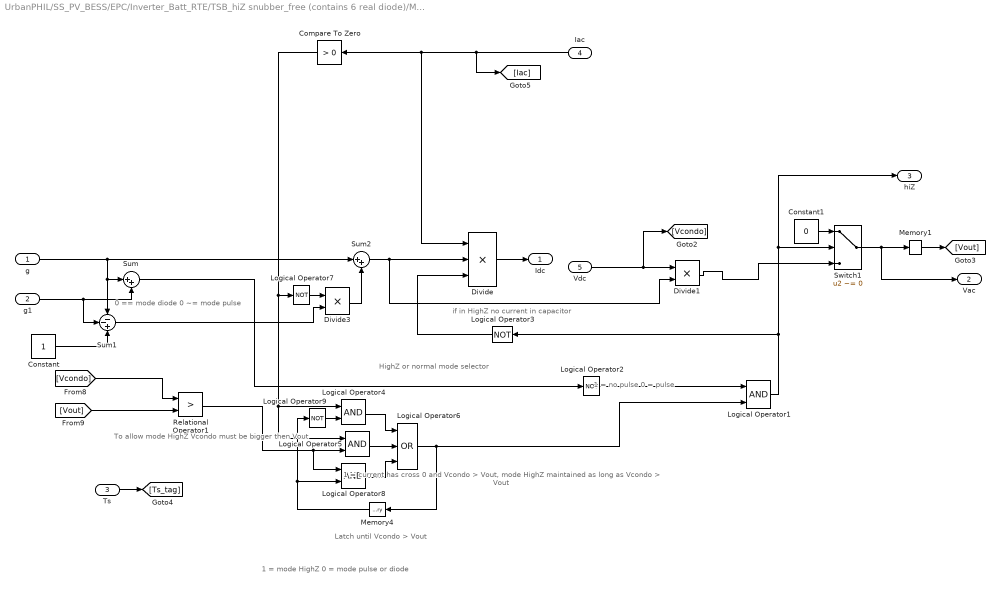
== system UrbanPHIL/SS_PV_BESS/EPC/Inverter_Batt_RTE/TSB_hiZ snubber_free (contains 6 real diode)/MMC_1P1/MMC_cell_Sfunction ==
  note: Latch until Vcondo > Vout
  note: 1 = mode HighZ
      | 0 = mode pulse or diode
  note: if in HighZ no current in capacitor
  note: 0 == mode diode
      | 0 ~= mode pulse
  note: 1 = current has cross 0 and
      | Vcondo > Vout, mode HighZ
      | maintained as long as Vcondo > Vout
  note: 1 = no pulse
      | 0 = pulse
  note: To allow mode HighZ
      | Vcondo must be bigger then
      | Vout
  note: HighZ or normal mode selector
  g : Inport
  g1 : Inport  Port=2
  Ts : Inport  Port=3
  Iac : Inport  Port=4
  Vdc : Inport  Port=5
  Compare To Zero : simulink/Logic and Bit Operations/Compare To Zero  relop=>  OutDataTypeStr=uint8
  Constant : Constant
  Constant1 : Constant  Value=0
  Divide : Product  Inputs=3
  Divide1 : Product
  Divide3 : Product
  Logical Operator{1,4..5,8} (4 alike) : Logic  AllPortsSameDT=off  OutDataTypeStr=boolean
  Logical Operator{2..3,7,9} (4 alike) : Logic  Operator=NOT  AllPortsSameDT=off  OutDataTypeStr=boolean
  Logical Operator6 : Logic  Operator=OR  Inputs=3  AllPortsSameDT=off  OutDataTypeStr=boolean
  Memory1 : Memory  InheritSampleTime=on
  Memory4 : Memory  InheritSampleTime=on
  Relational Operator1 : RelationalOperator  Operator=>  OutDataTypeStr=boolean
  Sum : Sum  Inputs=|++
  Sum1 : Sum  Inputs=--+
  Sum2 : Sum  Inputs=|++
  Switch1 : Switch  Criteria=u2 ~= 0
  Idc : Outport
  Vac : Outport  Port=2
  hiZ : Outport  Port=3
  wires:
  Memory1/1 -> [Vout]
  Divide3/1 -> Sum2/2
  Sum1/1 -> Divide3/2
  Constant/1 -> Sum1/3
  Logical Operator6/1 -> Memory4/1, Logical Operator1/2
  Logical Operator8/1 -> Logical Operator6/3
  Logical Operator5/1 -> Logical Operator6/2
  Logical Operator4/1 -> Logical Operator6/1
  Logical Operator9/1 -> Logical Operator4/2
  Relational Operator1/1 -> Logical Operator8/1, Logical Operator5/2
  Logical Operator7/1 -> Divide3/1
  Ts/1 -> [Ts_tag]
  g1/1 -> Sum1/2, Sum/2
  Logical Operator1/1 -> Logical Operator3/1, Switch1/2, hiZ/1
  [Vcondo] -> Relational Operator1/1
  Logical Operator3/1 -> Divide/3
  Logical Operator2/1 -> Logical Operator1/1
  [Vout] -> Relational Operator1/2
  Vdc/1 -> Divide1/1, [Vcondo]
  Iac/1 -> Compare To Zero/1, Divide/1, [Iac]
  Divide/1 -> Idc/1
  Compare To Zero/1 -> Logical Operator4/1, Logical Operator5/1, Logical Operator7/1
  Sum/1 -> Logical Operator2/1
  g/1 -> Sum1/1, Sum/1, Sum2/1
  Sum2/1 -> Divide1/2, Divide/2
  Divide1/1 -> Switch1/3
  Switch1/1 -> Memory1/1, Vac/1
  Memory4/1 -> Logical Operator8/2, Logical Operator9/1
  Constant1/1 -> Switch1/1

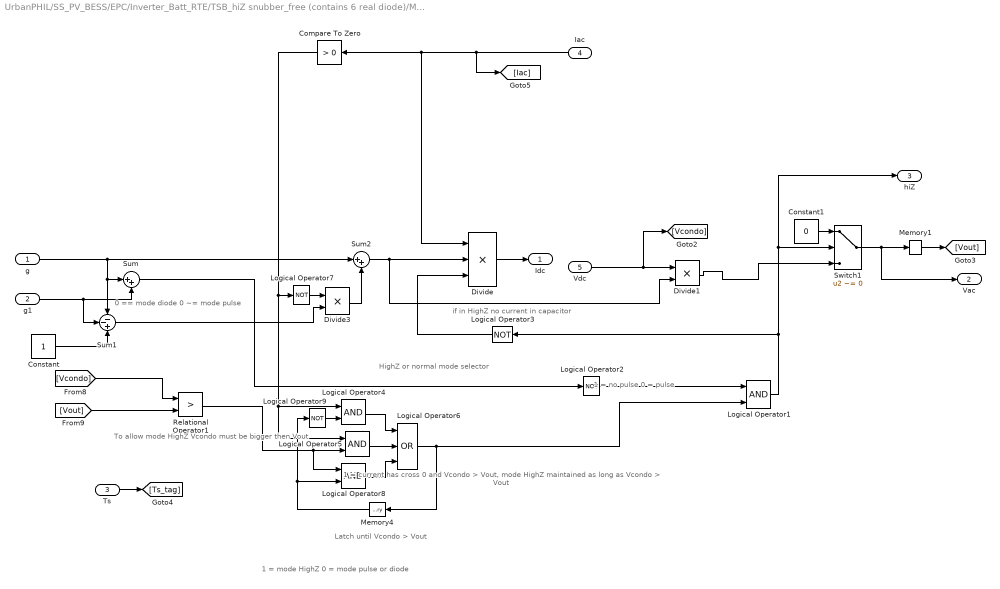
== system UrbanPHIL/SS_PV_BESS/EPC/Inverter_Batt_RTE/TSB_hiZ snubber_free (contains 6 real diode)/MMC_1P2/MMC_cell_Sfunction ==
  note: HighZ or normal mode selector
  note: To allow mode HighZ
      | Vcondo must be bigger then
      | Vout
  note: 1 = no pulse
      | 0 = pulse
  note: 1 = current has cross 0 and
      | Vcondo > Vout, mode HighZ
      | maintained as long as Vcondo > Vout
  note: 0 == mode diode
      | 0 ~= mode pulse
  note: if in HighZ no current in capacitor
  note: 1 = mode HighZ
      | 0 = mode pulse or diode
  note: Latch until Vcondo > Vout
  g : Inport
  g1 : Inport  Port=2
  Ts : Inport  Port=3
  Iac : Inport  Port=4
  Vdc : Inport  Port=5
  Compare To Zero : simulink/Logic and Bit Operations/Compare To Zero  relop=>  OutDataTypeStr=uint8
  Constant : Constant
  Constant1 : Constant  Value=0
  Divide : Product  Inputs=3
  Divide1 : Product
  Divide3 : Product
  Logical Operator{1,4..5,8} (4 alike) : Logic  AllPortsSameDT=off  OutDataTypeStr=boolean
  Logical Operator{2..3,7,9} (4 alike) : Logic  Operator=NOT  AllPortsSameDT=off  OutDataTypeStr=boolean
  Logical Operator6 : Logic  Operator=OR  Inputs=3  AllPortsSameDT=off  OutDataTypeStr=boolean
  Memory1 : Memory  InheritSampleTime=on
  Memory4 : Memory  InheritSampleTime=on
  Relational Operator1 : RelationalOperator  Operator=>  OutDataTypeStr=boolean
  Sum : Sum  Inputs=|++
  Sum1 : Sum  Inputs=--+
  Sum2 : Sum  Inputs=|++
  Switch1 : Switch  Criteria=u2 ~= 0
  Idc : Outport
  Vac : Outport  Port=2
  hiZ : Outport  Port=3
  wires:
  Constant1/1 -> Switch1/1
  Memory4/1 -> Logical Operator9/1, Logical Operator8/2
  Switch1/1 -> Vac/1, Memory1/1
  Divide1/1 -> Switch1/3
  Sum2/1 -> Divide/2, Divide1/2
  g/1 -> Sum2/1, Sum/1, Sum1/1
  Sum/1 -> Logical Operator2/1
  Compare To Zero/1 -> Logical Operator7/1, Logical Operator5/1, Logical Operator4/1
  Divide/1 -> Idc/1
  Iac/1 -> [Iac], Divide/1, Compare To Zero/1
  Vdc/1 -> [Vcondo], Divide1/1
  [Vout] -> Relational Operator1/2
  Logical Operator2/1 -> Logical Operator1/1
  Logical Operator3/1 -> Divide/3
  [Vcondo] -> Relational Operator1/1
  Logical Operator1/1 -> hiZ/1, Switch1/2, Logical Operator3/1
  g1/1 -> Sum/2, Sum1/2
  Ts/1 -> [Ts_tag]
  Logical Operator7/1 -> Divide3/1
  Relational Operator1/1 -> Logical Operator5/2, Logical Operator8/1
  Logical Operator9/1 -> Logical Operator4/2
  Logical Operator4/1 -> Logical Operator6/1
  Logical Operator5/1 -> Logical Operator6/2
  Logical Operator8/1 -> Logical Operator6/3
  Logical Operator6/1 -> Logical Operator1/2, Memory4/1
  Constant/1 -> Sum1/3
  Sum1/1 -> Divide3/2
  Divide3/1 -> Sum2/2
  Memory1/1 -> [Vout]

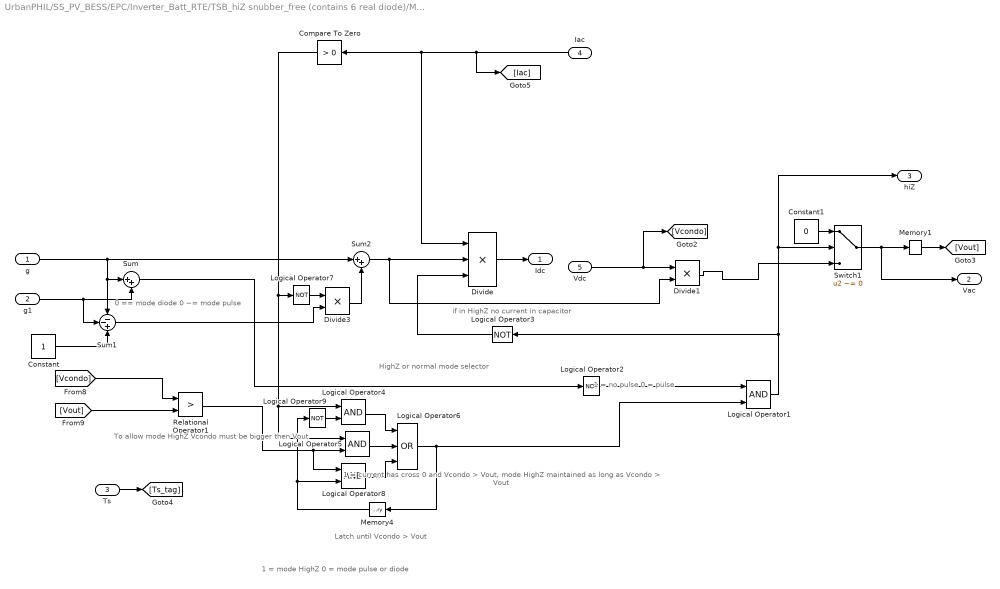
== system UrbanPHIL/SS_PV_BESS/EPC/Inverter_Batt_RTE/TSB_hiZ snubber_free (contains 6 real diode)/MMC_1P3/MMC_cell_Sfunction ==
  note: Latch until Vcondo > Vout
  note: 1 = mode HighZ
      | 0 = mode pulse or diode
  note: if in HighZ no current in capacitor
  note: 0 == mode diode
      | 0 ~= mode pulse
  note: 1 = current has cross 0 and
      | Vcondo > Vout, mode HighZ
      | maintained as long as Vcondo > Vout
  note: 1 = no pulse
      | 0 = pulse
  note: To allow mode HighZ
      | Vcondo must be bigger then
      | Vout
  note: HighZ or normal mode selector
  g : Inport
  g1 : Inport  Port=2
  Ts : Inport  Port=3
  Iac : Inport  Port=4
  Vdc : Inport  Port=5
  Compare To Zero : simulink/Logic and Bit Operations/Compare To Zero  relop=>  OutDataTypeStr=uint8
  Constant : Constant
  Constant1 : Constant  Value=0
  Divide : Product  Inputs=3
  Divide1 : Product
  Divide3 : Product
  Logical Operator{1,4..5,8} (4 alike) : Logic  AllPortsSameDT=off  OutDataTypeStr=boolean
  Logical Operator{2..3,7,9} (4 alike) : Logic  Operator=NOT  AllPortsSameDT=off  OutDataTypeStr=boolean
  Logical Operator6 : Logic  Operator=OR  Inputs=3  AllPortsSameDT=off  OutDataTypeStr=boolean
  Memory1 : Memory  InheritSampleTime=on
  Memory4 : Memory  InheritSampleTime=on
  Relational Operator1 : RelationalOperator  Operator=>  OutDataTypeStr=boolean
  Sum : Sum  Inputs=|++
  Sum1 : Sum  Inputs=--+
  Sum2 : Sum  Inputs=|++
  Switch1 : Switch  Criteria=u2 ~= 0
  Idc : Outport
  Vac : Outport  Port=2
  hiZ : Outport  Port=3
  wires:
  Memory1/1 -> [Vout]
  Divide3/1 -> Sum2/2
  Sum1/1 -> Divide3/2
  Constant/1 -> Sum1/3
  Logical Operator6/1 -> Memory4/1, Logical Operator1/2
  Logical Operator8/1 -> Logical Operator6/3
  Logical Operator5/1 -> Logical Operator6/2
  Logical Operator4/1 -> Logical Operator6/1
  Logical Operator9/1 -> Logical Operator4/2
  Relational Operator1/1 -> Logical Operator8/1, Logical Operator5/2
  Logical Operator7/1 -> Divide3/1
  Ts/1 -> [Ts_tag]
  g1/1 -> Sum1/2, Sum/2
  Logical Operator1/1 -> Logical Operator3/1, Switch1/2, hiZ/1
  [Vcondo] -> Relational Operator1/1
  Logical Operator3/1 -> Divide/3
  Logical Operator2/1 -> Logical Operator1/1
  [Vout] -> Relational Operator1/2
  Vdc/1 -> Divide1/1, [Vcondo]
  Iac/1 -> Compare To Zero/1, Divide/1, [Iac]
  Divide/1 -> Idc/1
  Compare To Zero/1 -> Logical Operator4/1, Logical Operator5/1, Logical Operator7/1
  Sum/1 -> Logical Operator2/1
  g/1 -> Sum1/1, Sum/1, Sum2/1
  Sum2/1 -> Divide1/2, Divide/2
  Divide1/1 -> Switch1/3
  Switch1/1 -> Memory1/1, Vac/1
  Memory4/1 -> Logical Operator8/2, Logical Operator9/1
  Constant1/1 -> Switch1/1
